simulink model "system_FFT_decoder_matlab"  (Simulink 8.3)
settings: Solver=ode45  StartTime=0.0  StopTime=0.06  RelTol=1e-3
settings Model: Creator=Vasilis  LastModifiedBy=Vasilis
settings OptimizationCC: ExpressionDepthLimit=2147483647
settings DebuggingCC: FcnCallInpInsideContextMsg=UseLocalSettings

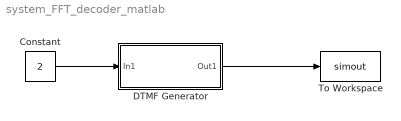
== system system_FFT_decoder_matlab ==
  Constant : Constant  Value=2
  DTMF Generator : Subsystem
  To Workspace : ToWorkspace  VariableName=simout  SaveFormat=Structure  SampleTime=-1
  wires:
  Constant/1 -> DTMF Generator/1(In1)
  DTMF Generator/1(Out1) -> To Workspace/1

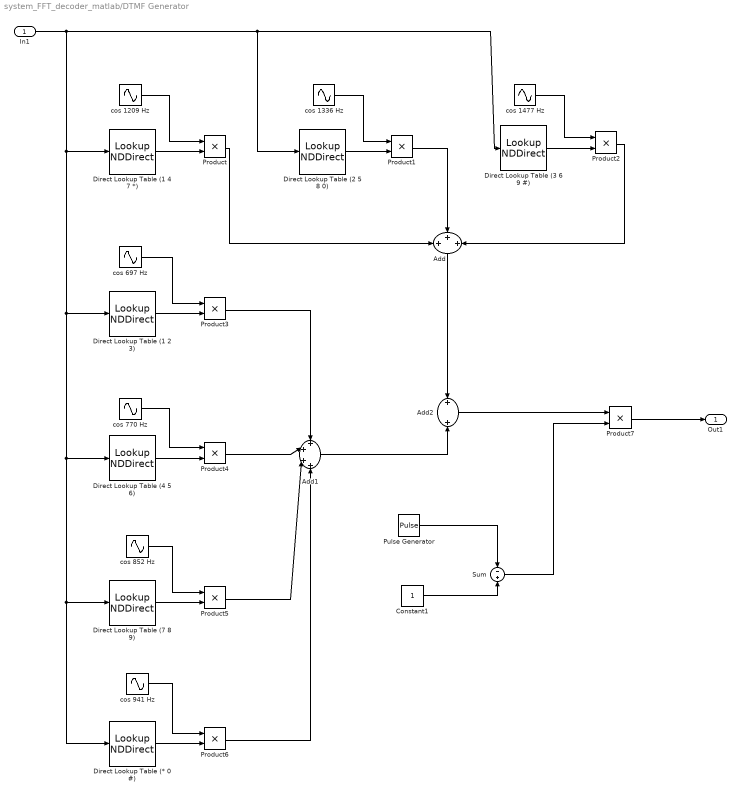
== system system_FFT_decoder_matlab/DTMF Generator ==
  In1 : Inport
  Add : Sum  Inputs=+++
  Add1 : Sum  Inputs=++++
  Add2 : Sum
  Constant1 : Constant
  Direct Lookup Table (* 0 #) : LookupNDDirect  NumberOfTableDimensions=1  Table=[1 0 0 0 0 0 0 0 0 0 1 1]
  Direct Lookup Table (1 2 3) : LookupNDDirect  NumberOfTableDimensions=1  Table=[0 1 1 1 0 0 0 0 0 0 0 0]
  Direct Lookup Table (1 4 7 *) : LookupNDDirect  NumberOfTableDimensions=1  Table=[0 1 0 0 1 0 0 1 0 0 1 0]
  Direct Lookup Table (2 5 8 0) : LookupNDDirect  NumberOfTableDimensions=1  Table=[1 0 1 0 0 1 0 0 1 0 0 0]
  Direct Lookup Table (3 6 9 #) : LookupNDDirect  NumberOfTableDimensions=1  Table=[0 0 0 1 0 0 1 0 0 1 0 1]
  Direct Lookup Table (4 5 6) : LookupNDDirect  NumberOfTableDimensions=1  Table=[0 0 0 0 1 1 1 0 0 0 0 0]
  Direct Lookup Table (7 8 9) : LookupNDDirect  NumberOfTableDimensions=1  Table=[0 0 0 0 0 0 0 1 1 1 0 0]
  Product{,1..7} (8 alike) : Product  RndMeth=Zero
  Pulse Generator : DiscretePulseGenerator  Period=479  PulseWidth=160  PhaseDelay=320  SampleTime=1/8000
  Sum : Sum  Inputs=-|+
  cos 1209 Hz : Sin  Frequency=7596  Phase=pi/2  SampleTime=1/8000
  cos 1336 Hz : Sin  Frequency=8394  Phase=pi/2  SampleTime=1/8000
  cos 1477 Hz : Sin  Frequency=9280  Phase=pi/2  SampleTime=1/8000
  cos 697 Hz : Sin  Frequency=4379  Phase=pi/2  SampleTime=1/8000
  cos 770 Hz : Sin  Frequency=4838  Phase=pi/2  SampleTime=1/8000
  cos 852 Hz : Sin  Frequency=5353  Phase=pi/2  SampleTime=1/8000
  cos 941 Hz : Sin  Frequency=5912  Phase=pi/2  SampleTime=1/8000
  Out1 : Outport
  wires:
  Direct Lookup Table (1 4 7 *)/1 -> Product/2
  In1/1 -> Direct Lookup Table (2 5 8 0)/1, Direct Lookup Table (3 6 9 #)/1, Direct Lookup Table (1 4 7 *)/1, Direct Lookup Table (1 2 3)/1, Direct Lookup Table (4 5 6)/1, Direct Lookup Table (7 8 9)/1, Direct Lookup Table (* 0 #)/1
  cos 1336 Hz/1 -> Product1/1
  Direct Lookup Table (2 5 8 0)/1 -> Product1/2
  cos 1477 Hz/1 -> Product2/1
  Direct Lookup Table (3 6 9 #)/1 -> Product2/2
  cos 697 Hz/1 -> Product3/1
  Direct Lookup Table (1 2 3)/1 -> Product3/2
  cos 770 Hz/1 -> Product4/1
  Direct Lookup Table (4 5 6)/1 -> Product4/2
  cos 852 Hz/1 -> Product5/1
  Direct Lookup Table (7 8 9)/1 -> Product5/2
  Product2/1 -> Add/3
  Product1/1 -> Add/2
  Product/1 -> Add/1
  Product3/1 -> Add1/1
  Product5/1 -> Add1/3
  Product4/1 -> Add1/2
  Add1/1 -> Add2/2
  Add/1 -> Add2/1
  cos 941 Hz/1 -> Product6/1
  Direct Lookup Table (* 0 #)/1 -> Product6/2
  Product6/1 -> Add1/4
  cos 1209 Hz/1 -> Product/1
  Constant1/1 -> Sum/2
  Pulse Generator/1 -> Sum/1
  Product7/1 -> Out1/1
  Add2/1 -> Product7/1
  Sum/1 -> Product7/2
